simulink model "aoc_ut"  (Simulink 8.1)
settings: Solver=FixedStepDiscrete  StartTime=0.0  StopTime=10.0  FixedStep=5E-3  RelTol=1e-3
libraries: siltestlib x4, aoc x1
settings Model: Creator=AT015086  LastModifiedBy=tescamilla
settings DataIOCC: SignalLoggingSaveFormat=Dataset
settings OptimizationCC: ExpressionDepthLimit=128
settings DebuggingCC: FcnCallInpInsideContextMsg=EnableAllAsError
settings GRTTargetCC: CombineOutputUpdateFcns=on  GRTInterface=off

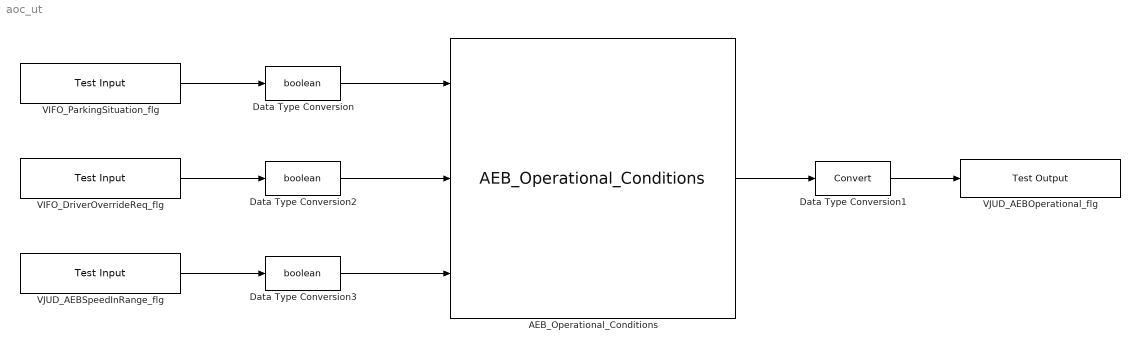
== system aoc_ut ==
  AEB_Operational_Conditions : aoc/AEB_Operational_Conditions
  Data Type Conversion : DataTypeConversion  OutDataTypeStr=boolean
  Data Type Conversion1 : DataTypeConversion
  Data Type Conversion2 : DataTypeConversion  OutDataTypeStr=boolean
  Data Type Conversion3 : DataTypeConversion  OutDataTypeStr=boolean
  VIFO_DriverOverrideReq_flg : siltestlib/Test Input  varname=VIFO_DriverOverrideReq_flg  sampletime=-1
  VIFO_ParkingSituation_flg : siltestlib/Test Input  varname=VIFO_ParkingSituation_flg  sampletime=-1
  VJUD_AEBOperational_flg : siltestlib/Test Output  varname=VJUD_AEBOperational_flg  sampletime=-1
  VJUD_AEBSpeedInRange_flg : siltestlib/Test Input  varname=VJUD_AEBSpeedInRange_flg  sampletime=-1
  wires:
  Data Type Conversion/1 -> AEB_Operational_Conditions/1
  VIFO_ParkingSituation_flg/1 -> Data Type Conversion/1
  AEB_Operational_Conditions/1 -> Data Type Conversion1/1
  Data Type Conversion1/1 -> VJUD_AEBOperational_flg/1
  VIFO_DriverOverrideReq_flg/1 -> Data Type Conversion2/1
  Data Type Conversion2/1 -> AEB_Operational_Conditions/2
  Data Type Conversion3/1 -> AEB_Operational_Conditions/3
  VJUD_AEBSpeedInRange_flg/1 -> Data Type Conversion3/1
